simulink model "SecRwLtStRclCmdSrvCal"  (R2018b)
settings: Solver=FixedStepDiscrete  StartTime=0.0  StopTime=10.0  FixedStep=0.01  RelTol=1e-3
undefined symbols (not defined in the file or in its folder): KeSMSwPosInvalidVal_Val, PowerMode1
settings Model: Creator=sn2xws  LastModifiedBy=sn2xws
settings Model: ModifiedHistory=|
  | 2024.5.6
  | V3.0.0 增加零重力电机
  | 2024.8.16 2LZero不动作问题修复
settings DataIOCC: SaveFormat=StructureWithTime
settings OptimizationCC: DefaultParameterBehavior=Inlined  EnhancedBackFolding=on  PassReuseOutputArgsAs=Individual arguments  ZeroExternalMemoryAtStartup=off  ZeroInternalMemoryAtStartup=off  OptimizeBlockOrder=speed  DifferentSizesBufferReuse=on  OptimizationCustomize=off
settings DebuggingCC: ParameterTunabilityLossMsg=error
settings ModelReferenceCC: ModelReferenceNumInstancesAllowed=Single
settings SFSimCC: MATLABDynamicMemAlloc=off
settings RTWCC: SystemTargetFile=autosar.tlc  GenCodeOnly=on  TemplateMakefile=ert_default_tmf  Description=AUTOSAR  GenerateReport=on  IncludeHyperlinkInReport=on  LaunchReport=on  GenerateTraceInfo=on  GenerateTraceReport=on  GenerateTraceReportSl=on  GenerateTraceReportSf=on  GenerateTraceReportEml=on  GenerateCodeMetricsReport=on
settings CodeAppCC: ForceParamTrailComments=on  IgnoreCustomStorageClasses=off  OperatorAnnotations=on  SimulinkDataObjDesc=on  SFDataObjDesc=on  InsertBlockDesc=on
settings STFCustomTargetCC: TargetLangStandard=C99 (ISO)  MultiwordLength=256  ParMdlRefBuildCompliant=on  CompOptLevelCompliant=on  IncludeMdlTerminateFcn=off  CombineOutputUpdateFcns=on  SuppressErrorStatus=on  ERTCustomFileBanners=on  SupportNonFinite=off  SupportComplex=off  SupportContinuousTime=off  SupportNonInlinedSFcns=off  RemoveResetFunc=on  MATLABClassNameForMDSCustomization=Simulink.SoftwareTarget.ERTCustomization  AutosarCompliant=on  UseToolchainInfoCompliant=on  LookupTableObjectStructAxisOrder=2,1,3,4,...  LUTObjectStructOrderEvenSpacing=Size,Table,Breakpoints  SystemTargetFile=autosar.tlc
settings ERTTargetCC: TargetLangStandard=C99 (ISO)  ConcurrentExecutionCompliant=off  IncludeMdlTerminateFcn=off  SuppressErrorStatus=on  SupportNonFinite=off  SupportComplex=off  ModelStepFunctionPrototypeControlCompliant=off  CPPClassGenCompliant=off  AutosarCompliant=on  LookupTableObjectStructAxisOrder=2,1,3,4,...  LUTObjectStructOrderEvenSpacing=Size,Table,Breakpoints  InlinedParameterPlacement=NonHierarchical  ERTCustomFileTemplate=example_file_process.tlc  ERTFilePackagingFormat=Compact

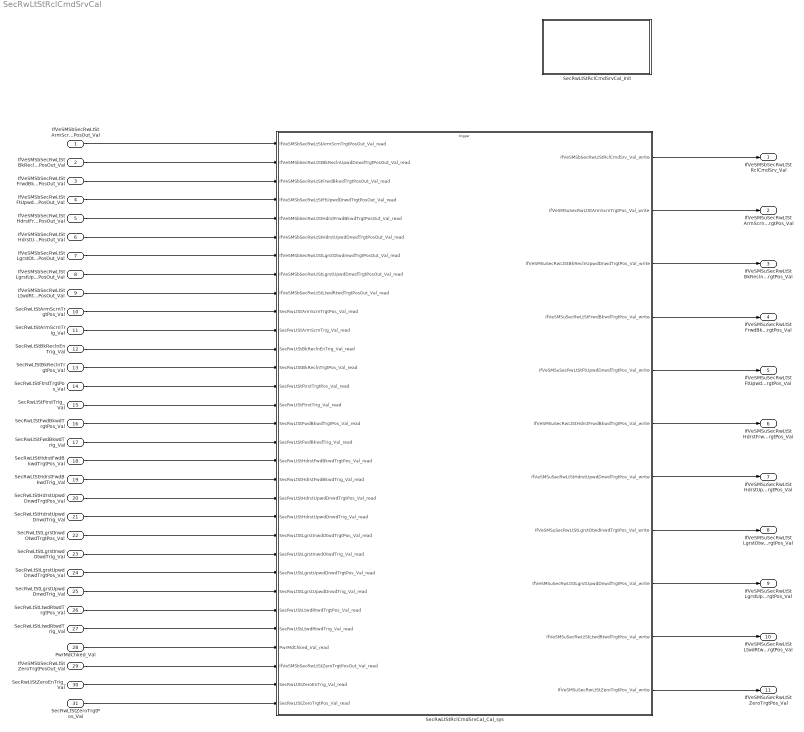
== system SecRwLtStRclCmdSrvCal ==
  IfVeSMSbSecRwLtStArmScrnTrgtPosOut_Val : Inport  OutDataTypeStr=boolean  PortDimensions=1
  IfVeSMSbSecRwLtStBkReclnUpwdDnwdTrgtPosOut_Val : Inport  Port=2  OutDataTypeStr=boolean  PortDimensions=1
  IfVeSMSbSecRwLtStFrwdBkwdTrgtPosOut_Val : Inport  Port=3  OutDataTypeStr=boolean  PortDimensions=1
  IfVeSMSbSecRwLtStFtUpwdDnwdTrgtPosOut_Val : Inport  Port=4  OutDataTypeStr=boolean  PortDimensions=1
  IfVeSMSbSecRwLtStHdrstFrwdBkwdTrgtPosOut_Val : Inport  Port=5  OutDataTypeStr=boolean  PortDimensions=1
  IfVeSMSbSecRwLtStHdrstUpwdDnwdTrgtPosOut_Val : Inport  Port=6  OutDataTypeStr=boolean  PortDimensions=1
  IfVeSMSbSecRwLtStLgrstOtwdInwdTrgtPosOut_Val : Inport  Port=7  OutDataTypeStr=boolean  PortDimensions=1
  IfVeSMSbSecRwLtStLgrstUpwdDnwdTrgtPosOut_Val : Inport  Port=8  OutDataTypeStr=boolean  PortDimensions=1
  IfVeSMSbSecRwLtStLtwdRtwdTrgtPosOut_Val : Inport  Port=9  OutDataTypeStr=boolean  PortDimensions=1
  SecRwLtStArmScrnTrgtPos_Val : Inport  Port=10  OutDataTypeStr=uint16  PortDimensions=1
  SecRwLtStArmScrnTrig_Val : Inport  Port=11  OutDataTypeStr=boolean  PortDimensions=1
  SecRwLtStBkReclnEnTrig_Val : Inport  Port=12  OutDataTypeStr=boolean  PortDimensions=1
  SecRwLtStBkReclnTrgtPos_Val : Inport  Port=13  OutDataTypeStr=uint16  PortDimensions=1
  SecRwLtStFtrstTrgtPos_Val : Inport  Port=14  OutDataTypeStr=uint16  PortDimensions=1
  SecRwLtStFtrstTrig_Val : Inport  Port=15  OutDataTypeStr=boolean  PortDimensions=1
  SecRwLtStFwdBkwdTrgtPos_Val : Inport  Port=16  OutDataTypeStr=uint16  PortDimensions=1
  SecRwLtStFwdBkwdTrig_Val : Inport  Port=17  OutDataTypeStr=boolean  PortDimensions=1
  SecRwLtStHdrstFwdBkwdTrgtPos_Val : Inport  Port=18  OutDataTypeStr=uint16  PortDimensions=1
  SecRwLtStHdrstFwdBkwdTrig_Val : Inport  Port=19  OutDataTypeStr=boolean  PortDimensions=1
  SecRwLtStHdrstUpwdDnwdTrgtPos_Val : Inport  Port=20  OutDataTypeStr=uint16  PortDimensions=1
  SecRwLtStHdrstUpwdDnwdTrig_Val : Inport  Port=21  OutDataTypeStr=boolean  PortDimensions=1
  SecRwLtStLgrstInwdOtwdTrgtPos_Val : Inport  Port=22  OutDataTypeStr=uint16  PortDimensions=1
  SecRwLtStLgrstInwdOtwdTrig_Val : Inport  Port=23  OutDataTypeStr=boolean  PortDimensions=1
  SecRwLtStLgrstUpwdDnwdTrgtPos_Val : Inport  Port=24  OutDataTypeStr=uint16  PortDimensions=1
  SecRwLtStLgrstUpwdDnwdTrig_Val : Inport  Port=25  OutDataTypeStr=boolean  PortDimensions=1
  SecRwLtStLtwdRtwdTrgtPos_Val : Inport  Port=26  OutDataTypeStr=uint16  PortDimensions=1
  SecRwLtStLtwdRtwdTrig_Val : Inport  Port=27  OutDataTypeStr=boolean  PortDimensions=1
  PwrMdChked_Val : Inport  Port=28  OutDataTypeStr=Enum: PowerMode1  PortDimensions=1
  IfVeSMSbSecRwLtStZeroTrgtPosOut_Val : Inport  Port=29  OutDataTypeStr=boolean  PortDimensions=1
  SecRwLtStZeroEnTrig_Val : Inport  Port=30  OutDataTypeStr=boolean  PortDimensions=1
  SecRwLtStZeroTrgtPos_Val : Inport  Port=31  OutDataTypeStr=uint16  PortDimensions=1
  SecRwLtStRclCmdSrvCal_Cal_sys : Subsystem
  SecRwLtStRclCmdSrvCal_Init : Subsystem
  IfVeSMSbSecRwLtStRclCmdSrv_Val : Outport  OutDataTypeStr=boolean  PortDimensions=1
  IfVeSMSuSecRwLtStArmScrnTrgtPos_Val : Outport  Port=2  OutDataTypeStr=uint16  PortDimensions=1
  IfVeSMSuSecRwLtStBkReclnUpwdDnwdTrgtPos_Val : Outport  Port=3  OutDataTypeStr=uint16  PortDimensions=1
  IfVeSMSuSecRwLtStFrwdBkwdTrgtPos_Val : Outport  Port=4  OutDataTypeStr=uint16  PortDimensions=1
  IfVeSMSuSecRwLtStFtUpwdDnwdTrgtPos_Val : Outport  Port=5  OutDataTypeStr=uint16  PortDimensions=1
  IfVeSMSuSecRwLtStHdrstFrwdBkwdTrgtPos_Val : Outport  Port=6  OutDataTypeStr=uint16  PortDimensions=1
  IfVeSMSuSecRwLtStHdrstUpwdDnwdTrgtPos_Val : Outport  Port=7  OutDataTypeStr=uint16  PortDimensions=1
  IfVeSMSuSecRwLtStLgrstOtwdInwdTrgtPos_Val : Outport  Port=8  OutDataTypeStr=uint16  PortDimensions=1
  IfVeSMSuSecRwLtStLgrstUpwdDnwdTrgtPos_Val : Outport  Port=9  OutDataTypeStr=uint16  PortDimensions=1
  IfVeSMSuSecRwLtStLtwdRtwdTrgtPos_Val : Outport  Port=10  OutDataTypeStr=uint16  PortDimensions=1
  IfVeSMSuSecRwLtStZeroTrgtPos_Val : Outport  Port=11  OutDataTypeStr=uint16  PortDimensions=1
  wires:
  IfVeSMSbSecRwLtStArmScrnTrgtPosOut_Val/1 -> SecRwLtStRclCmdSrvCal_Cal_sys/1(IfVeSMSbSecRwLtStArmScrnTrgtPosOut_Val_read)
  IfVeSMSbSecRwLtStBkReclnUpwdDnwdTrgtPosOut_Val/1 -> SecRwLtStRclCmdSrvCal_Cal_sys/2(IfVeSMSbSecRwLtStBkReclnUpwdDnwdTrgtPosOut_Val_read)
  IfVeSMSbSecRwLtStFrwdBkwdTrgtPosOut_Val/1 -> SecRwLtStRclCmdSrvCal_Cal_sys/3(IfVeSMSbSecRwLtStFrwdBkwdTrgtPosOut_Val_read)
  IfVeSMSbSecRwLtStFtUpwdDnwdTrgtPosOut_Val/1 -> SecRwLtStRclCmdSrvCal_Cal_sys/4(IfVeSMSbSecRwLtStFtUpwdDnwdTrgtPosOut_Val_read)
  IfVeSMSbSecRwLtStHdrstFrwdBkwdTrgtPosOut_Val/1 -> SecRwLtStRclCmdSrvCal_Cal_sys/5(IfVeSMSbSecRwLtStHdrstFrwdBkwdTrgtPosOut_Val_read)
  IfVeSMSbSecRwLtStHdrstUpwdDnwdTrgtPosOut_Val/1 -> SecRwLtStRclCmdSrvCal_Cal_sys/6(IfVeSMSbSecRwLtStHdrstUpwdDnwdTrgtPosOut_Val_read)
  IfVeSMSbSecRwLtStLgrstOtwdInwdTrgtPosOut_Val/1 -> SecRwLtStRclCmdSrvCal_Cal_sys/7(IfVeSMSbSecRwLtStLgrstOtwdInwdTrgtPosOut_Val_read)
  IfVeSMSbSecRwLtStLgrstUpwdDnwdTrgtPosOut_Val/1 -> SecRwLtStRclCmdSrvCal_Cal_sys/8(IfVeSMSbSecRwLtStLgrstUpwdDnwdTrgtPosOut_Val_read)
  IfVeSMSbSecRwLtStLtwdRtwdTrgtPosOut_Val/1 -> SecRwLtStRclCmdSrvCal_Cal_sys/9(IfVeSMSbSecRwLtStLtwdRtwdTrgtPosOut_Val_read)
  SecRwLtStArmScrnTrgtPos_Val/1 -> SecRwLtStRclCmdSrvCal_Cal_sys/10(SecRwLtStArmScrnTrgtPos_Val_read)
  SecRwLtStArmScrnTrig_Val/1 -> SecRwLtStRclCmdSrvCal_Cal_sys/11(SecRwLtStArmScrnTrig_Val_read)
  SecRwLtStBkReclnEnTrig_Val/1 -> SecRwLtStRclCmdSrvCal_Cal_sys/12(SecRwLtStBkReclnEnTrig_Val_read)
  SecRwLtStBkReclnTrgtPos_Val/1 -> SecRwLtStRclCmdSrvCal_Cal_sys/13(SecRwLtStBkReclnTrgtPos_Val_read)
  SecRwLtStFtrstTrgtPos_Val/1 -> SecRwLtStRclCmdSrvCal_Cal_sys/14(SecRwLtStFtrstTrgtPos_Val_read)
  SecRwLtStFtrstTrig_Val/1 -> SecRwLtStRclCmdSrvCal_Cal_sys/15(SecRwLtStFtrstTrig_Val_read)
  SecRwLtStFwdBkwdTrgtPos_Val/1 -> SecRwLtStRclCmdSrvCal_Cal_sys/16(SecRwLtStFwdBkwdTrgtPos_Val_read)
  SecRwLtStFwdBkwdTrig_Val/1 -> SecRwLtStRclCmdSrvCal_Cal_sys/17(SecRwLtStFwdBkwdTrig_Val_read)
  SecRwLtStHdrstFwdBkwdTrgtPos_Val/1 -> SecRwLtStRclCmdSrvCal_Cal_sys/18(SecRwLtStHdrstFwdBkwdTrgtPos_Val_read)
  SecRwLtStHdrstFwdBkwdTrig_Val/1 -> SecRwLtStRclCmdSrvCal_Cal_sys/19(SecRwLtStHdrstFwdBkwdTrig_Val_read)
  SecRwLtStHdrstUpwdDnwdTrgtPos_Val/1 -> SecRwLtStRclCmdSrvCal_Cal_sys/20(SecRwLtStHdrstUpwdDnwdTrgtPos_Val_read)
  SecRwLtStHdrstUpwdDnwdTrig_Val/1 -> SecRwLtStRclCmdSrvCal_Cal_sys/21(SecRwLtStHdrstUpwdDnwdTrig_Val_read)
  SecRwLtStLgrstInwdOtwdTrgtPos_Val/1 -> SecRwLtStRclCmdSrvCal_Cal_sys/22(SecRwLtStLgrstInwdOtwdTrgtPos_Val_read)
  SecRwLtStLgrstInwdOtwdTrig_Val/1 -> SecRwLtStRclCmdSrvCal_Cal_sys/23(SecRwLtStLgrstInwdOtwdTrig_Val_read)
  SecRwLtStLgrstUpwdDnwdTrgtPos_Val/1 -> SecRwLtStRclCmdSrvCal_Cal_sys/24(SecRwLtStLgrstUpwdDnwdTrgtPos_Val_read)
  SecRwLtStLgrstUpwdDnwdTrig_Val/1 -> SecRwLtStRclCmdSrvCal_Cal_sys/25(SecRwLtStLgrstUpwdDnwdTrig_Val_read)
  SecRwLtStLtwdRtwdTrgtPos_Val/1 -> SecRwLtStRclCmdSrvCal_Cal_sys/26(SecRwLtStLtwdRtwdTrgtPos_Val_read)
  SecRwLtStLtwdRtwdTrig_Val/1 -> SecRwLtStRclCmdSrvCal_Cal_sys/27(SecRwLtStLtwdRtwdTrig_Val_read)
  SecRwLtStRclCmdSrvCal_Cal_sys/1(IfVeSMSbSecRwLtStRclCmdSrv_Val_write) -> IfVeSMSbSecRwLtStRclCmdSrv_Val/1
  SecRwLtStRclCmdSrvCal_Cal_sys/2(IfVeSMSuSecRwLtStArmScrnTrgtPos_Val_write) -> IfVeSMSuSecRwLtStArmScrnTrgtPos_Val/1
  SecRwLtStRclCmdSrvCal_Cal_sys/3(IfVeSMSuSecRwLtStBkReclnUpwdDnwdTrgtPos_Val_write) -> IfVeSMSuSecRwLtStBkReclnUpwdDnwdTrgtPos_Val/1
  SecRwLtStRclCmdSrvCal_Cal_sys/4(IfVeSMSuSecRwLtStFrwdBkwdTrgtPos_Val_write) -> IfVeSMSuSecRwLtStFrwdBkwdTrgtPos_Val/1
  SecRwLtStRclCmdSrvCal_Cal_sys/5(IfVeSMSuSecRwLtStFtUpwdDnwdTrgtPos_Val_write) -> IfVeSMSuSecRwLtStFtUpwdDnwdTrgtPos_Val/1
  SecRwLtStRclCmdSrvCal_Cal_sys/6(IfVeSMSuSecRwLtStHdrstFrwdBkwdTrgtPos_Val_write) -> IfVeSMSuSecRwLtStHdrstFrwdBkwdTrgtPos_Val/1
  SecRwLtStRclCmdSrvCal_Cal_sys/7(IfVeSMSuSecRwLtStHdrstUpwdDnwdTrgtPos_Val_write) -> IfVeSMSuSecRwLtStHdrstUpwdDnwdTrgtPos_Val/1
  SecRwLtStRclCmdSrvCal_Cal_sys/8(IfVeSMSuSecRwLtStLgrstOtwdInwdTrgtPos_Val_write) -> IfVeSMSuSecRwLtStLgrstOtwdInwdTrgtPos_Val/1
  SecRwLtStRclCmdSrvCal_Cal_sys/9(IfVeSMSuSecRwLtStLgrstUpwdDnwdTrgtPos_Val_write) -> IfVeSMSuSecRwLtStLgrstUpwdDnwdTrgtPos_Val/1
  SecRwLtStRclCmdSrvCal_Cal_sys/10(IfVeSMSuSecRwLtStLtwdRtwdTrgtPos_Val_write) -> IfVeSMSuSecRwLtStLtwdRtwdTrgtPos_Val/1
  PwrMdChked_Val/1 -> SecRwLtStRclCmdSrvCal_Cal_sys/28(PwrMdChked_Val_read)
  IfVeSMSbSecRwLtStZeroTrgtPosOut_Val/1 -> SecRwLtStRclCmdSrvCal_Cal_sys/29(IfVeSMSbSecRwLtStZeroTrgtPosOut_Val_read)
  SecRwLtStZeroEnTrig_Val/1 -> SecRwLtStRclCmdSrvCal_Cal_sys/30(SecRwLtStZeroEnTrig_Val_read)
  SecRwLtStZeroTrgtPos_Val/1 -> SecRwLtStRclCmdSrvCal_Cal_sys/31(SecRwLtStZeroTrgtPos_Val_read)
  SecRwLtStRclCmdSrvCal_Cal_sys/11(IfVeSMSuSecRwLtStZeroTrgtPos_Val_write) -> IfVeSMSuSecRwLtStZeroTrgtPos_Val/1

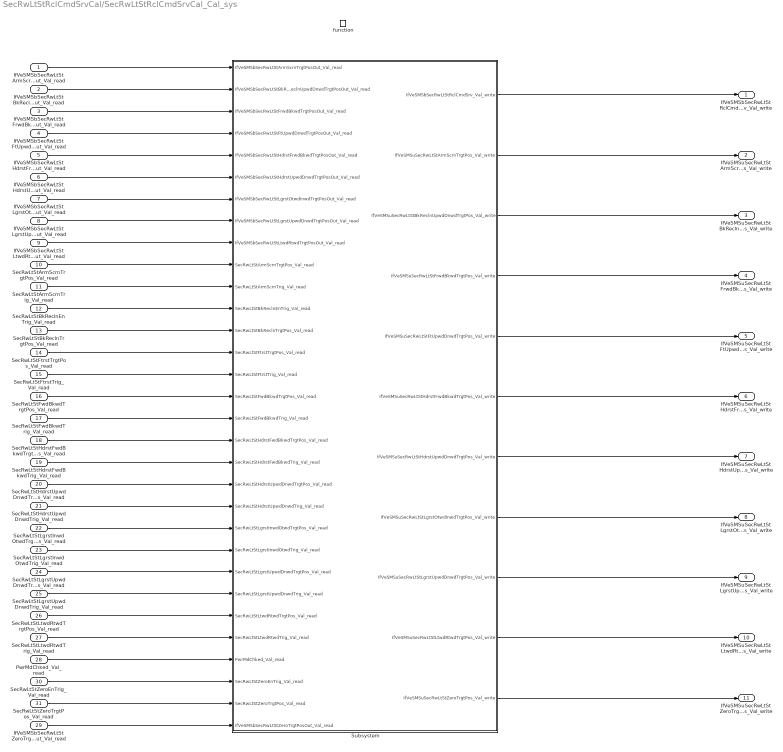
== system SecRwLtStRclCmdSrvCal/SecRwLtStRclCmdSrvCal_Cal_sys ==
  IfVeSMSbSecRwLtStArmScrnTrgtPosOut_Val_read : Inport
  IfVeSMSbSecRwLtStBkReclnUpwdDnwdTrgtPosOut_Val_read : Inport  Port=2
  IfVeSMSbSecRwLtStFrwdBkwdTrgtPosOut_Val_read : Inport  Port=3
  IfVeSMSbSecRwLtStFtUpwdDnwdTrgtPosOut_Val_read : Inport  Port=4
  IfVeSMSbSecRwLtStHdrstFrwdBkwdTrgtPosOut_Val_read : Inport  Port=5
  IfVeSMSbSecRwLtStHdrstUpwdDnwdTrgtPosOut_Val_read : Inport  Port=6
  IfVeSMSbSecRwLtStLgrstOtwdInwdTrgtPosOut_Val_read : Inport  Port=7
  IfVeSMSbSecRwLtStLgrstUpwdDnwdTrgtPosOut_Val_read : Inport  Port=8
  IfVeSMSbSecRwLtStLtwdRtwdTrgtPosOut_Val_read : Inport  Port=9
  SecRwLtStArmScrnTrgtPos_Val_read : Inport  Port=10
  SecRwLtStArmScrnTrig_Val_read : Inport  Port=11
  SecRwLtStBkReclnEnTrig_Val_read : Inport  Port=12
  SecRwLtStBkReclnTrgtPos_Val_read : Inport  Port=13
  SecRwLtStFtrstTrgtPos_Val_read : Inport  Port=14
  SecRwLtStFtrstTrig_Val_read : Inport  Port=15
  SecRwLtStFwdBkwdTrgtPos_Val_read : Inport  Port=16
  SecRwLtStFwdBkwdTrig_Val_read : Inport  Port=17
  SecRwLtStHdrstFwdBkwdTrgtPos_Val_read : Inport  Port=18
  SecRwLtStHdrstFwdBkwdTrig_Val_read : Inport  Port=19
  SecRwLtStHdrstUpwdDnwdTrgtPos_Val_read : Inport  Port=20
  SecRwLtStHdrstUpwdDnwdTrig_Val_read : Inport  Port=21
  SecRwLtStLgrstInwdOtwdTrgtPos_Val_read : Inport  Port=22
  SecRwLtStLgrstInwdOtwdTrig_Val_read : Inport  Port=23
  SecRwLtStLgrstUpwdDnwdTrgtPos_Val_read : Inport  Port=24
  SecRwLtStLgrstUpwdDnwdTrig_Val_read : Inport  Port=25
  SecRwLtStLtwdRtwdTrgtPos_Val_read : Inport  Port=26
  SecRwLtStLtwdRtwdTrig_Val_read : Inport  Port=27
  PwrMdChked_Val_read : Inport  Port=28
  IfVeSMSbSecRwLtStZeroTrgtPosOut_Val_read : Inport  Port=29
  SecRwLtStZeroEnTrig_Val_read : Inport  Port=30
  SecRwLtStZeroTrgtPos_Val_read : Inport  Port=31
  function : TriggerPort  TriggerType=function-call  IsSimulinkFunction=on  FunctionName=SecRwLtStRclCmdSrvCal_Cal  VariantControl=(inherit)
  Subsystem : Subsystem
  IfVeSMSbSecRwLtStRclCmdSrv_Val_write : Outport
      settings: EnsureOutportIsVirtual=on
  IfVeSMSuSecRwLtStArmScrnTrgtPos_Val_write : Outport  Port=2
      settings: EnsureOutportIsVirtual=on
  IfVeSMSuSecRwLtStBkReclnUpwdDnwdTrgtPos_Val_write : Outport  Port=3
      settings: EnsureOutportIsVirtual=on
  IfVeSMSuSecRwLtStFrwdBkwdTrgtPos_Val_write : Outport  Port=4
      settings: EnsureOutportIsVirtual=on
  IfVeSMSuSecRwLtStFtUpwdDnwdTrgtPos_Val_write : Outport  Port=5
      settings: EnsureOutportIsVirtual=on
  IfVeSMSuSecRwLtStHdrstFrwdBkwdTrgtPos_Val_write : Outport  Port=6
      settings: EnsureOutportIsVirtual=on
  IfVeSMSuSecRwLtStHdrstUpwdDnwdTrgtPos_Val_write : Outport  Port=7
      settings: EnsureOutportIsVirtual=on
  IfVeSMSuSecRwLtStLgrstOtwdInwdTrgtPos_Val_write : Outport  Port=8
      settings: EnsureOutportIsVirtual=on
  IfVeSMSuSecRwLtStLgrstUpwdDnwdTrgtPos_Val_write : Outport  Port=9
      settings: EnsureOutportIsVirtual=on
  IfVeSMSuSecRwLtStLtwdRtwdTrgtPos_Val_write : Outport  Port=10
      settings: EnsureOutportIsVirtual=on
  IfVeSMSuSecRwLtStZeroTrgtPos_Val_write : Outport  Port=11
      settings: EnsureOutportIsVirtual=on
  wires:
  IfVeSMSbSecRwLtStHdrstUpwdDnwdTrgtPosOut_Val_read/1 -> Subsystem/6(IfVeSMSbSecRwLtStHdrstUpwdDnwdTrgtPosOut_Val_read)
  IfVeSMSbSecRwLtStLgrstOtwdInwdTrgtPosOut_Val_read/1 -> Subsystem/7(IfVeSMSbSecRwLtStLgrstOtwdInwdTrgtPosOut_Val_read)
  IfVeSMSbSecRwLtStLgrstUpwdDnwdTrgtPosOut_Val_read/1 -> Subsystem/8(IfVeSMSbSecRwLtStLgrstUpwdDnwdTrgtPosOut_Val_read)
  IfVeSMSbSecRwLtStFtUpwdDnwdTrgtPosOut_Val_read/1 -> Subsystem/4(IfVeSMSbSecRwLtStFtUpwdDnwdTrgtPosOut_Val_read)
  IfVeSMSbSecRwLtStHdrstFrwdBkwdTrgtPosOut_Val_read/1 -> Subsystem/5(IfVeSMSbSecRwLtStHdrstFrwdBkwdTrgtPosOut_Val_read)
  IfVeSMSbSecRwLtStLtwdRtwdTrgtPosOut_Val_read/1 -> Subsystem/9(IfVeSMSbSecRwLtStLtwdRtwdTrgtPosOut_Val_read)
  SecRwLtStArmScrnTrgtPos_Val_read/1 -> Subsystem/10(SecRwLtStArmScrnTrgtPos_Val_read)
  IfVeSMSbSecRwLtStArmScrnTrgtPosOut_Val_read/1 -> Subsystem/1(IfVeSMSbSecRwLtStArmScrnTrgtPosOut_Val_read)
  IfVeSMSbSecRwLtStBkReclnUpwdDnwdTrgtPosOut_Val_read/1 -> Subsystem/2(IfVeSMSbSecRwLtStBkReclnUpwdDnwdTrgtPosOut_Val_read)
  IfVeSMSbSecRwLtStFrwdBkwdTrgtPosOut_Val_read/1 -> Subsystem/3(IfVeSMSbSecRwLtStFrwdBkwdTrgtPosOut_Val_read)
  SecRwLtStArmScrnTrig_Val_read/1 -> Subsystem/11(SecRwLtStArmScrnTrig_Val_read)
  SecRwLtStBkReclnEnTrig_Val_read/1 -> Subsystem/12(SecRwLtStBkReclnEnTrig_Val_read)
  SecRwLtStBkReclnTrgtPos_Val_read/1 -> Subsystem/13(SecRwLtStBkReclnTrgtPos_Val_read)
  SecRwLtStFtrstTrgtPos_Val_read/1 -> Subsystem/14(SecRwLtStFtrstTrgtPos_Val_read)
  SecRwLtStFtrstTrig_Val_read/1 -> Subsystem/15(SecRwLtStFtrstTrig_Val_read)
  SecRwLtStFwdBkwdTrgtPos_Val_read/1 -> Subsystem/16(SecRwLtStFwdBkwdTrgtPos_Val_read)
  SecRwLtStFwdBkwdTrig_Val_read/1 -> Subsystem/17(SecRwLtStFwdBkwdTrig_Val_read)
  SecRwLtStHdrstFwdBkwdTrgtPos_Val_read/1 -> Subsystem/18(SecRwLtStHdrstFwdBkwdTrgtPos_Val_read)
  SecRwLtStHdrstFwdBkwdTrig_Val_read/1 -> Subsystem/19(SecRwLtStHdrstFwdBkwdTrig_Val_read)
  SecRwLtStHdrstUpwdDnwdTrgtPos_Val_read/1 -> Subsystem/20(SecRwLtStHdrstUpwdDnwdTrgtPos_Val_read)
  SecRwLtStHdrstUpwdDnwdTrig_Val_read/1 -> Subsystem/21(SecRwLtStHdrstUpwdDnwdTrig_Val_read)
  SecRwLtStLgrstInwdOtwdTrgtPos_Val_read/1 -> Subsystem/22(SecRwLtStLgrstInwdOtwdTrgtPos_Val_read)
  SecRwLtStLgrstInwdOtwdTrig_Val_read/1 -> Subsystem/23(SecRwLtStLgrstInwdOtwdTrig_Val_read)
  SecRwLtStLgrstUpwdDnwdTrgtPos_Val_read/1 -> Subsystem/24(SecRwLtStLgrstUpwdDnwdTrgtPos_Val_read)
  SecRwLtStLgrstUpwdDnwdTrig_Val_read/1 -> Subsystem/25(SecRwLtStLgrstUpwdDnwdTrig_Val_read)
  SecRwLtStLtwdRtwdTrgtPos_Val_read/1 -> Subsystem/26(SecRwLtStLtwdRtwdTrgtPos_Val_read)
  SecRwLtStLtwdRtwdTrig_Val_read/1 -> Subsystem/27(SecRwLtStLtwdRtwdTrig_Val_read)
  Subsystem/1(IfVeSMSbSecRwLtStRclCmdSrv_Val_write) -> IfVeSMSbSecRwLtStRclCmdSrv_Val_write/1
  Subsystem/2(IfVeSMSuSecRwLtStArmScrnTrgtPos_Val_write) -> IfVeSMSuSecRwLtStArmScrnTrgtPos_Val_write/1
  Subsystem/3(IfVeSMSuSecRwLtStBkReclnUpwdDnwdTrgtPos_Val_write) -> IfVeSMSuSecRwLtStBkReclnUpwdDnwdTrgtPos_Val_write/1
  Subsystem/4(IfVeSMSuSecRwLtStFrwdBkwdTrgtPos_Val_write) -> IfVeSMSuSecRwLtStFrwdBkwdTrgtPos_Val_write/1
  Subsystem/5(IfVeSMSuSecRwLtStFtUpwdDnwdTrgtPos_Val_write) -> IfVeSMSuSecRwLtStFtUpwdDnwdTrgtPos_Val_write/1
  Subsystem/6(IfVeSMSuSecRwLtStHdrstFrwdBkwdTrgtPos_Val_write) -> IfVeSMSuSecRwLtStHdrstFrwdBkwdTrgtPos_Val_write/1
  Subsystem/7(IfVeSMSuSecRwLtStHdrstUpwdDnwdTrgtPos_Val_write) -> IfVeSMSuSecRwLtStHdrstUpwdDnwdTrgtPos_Val_write/1
  Subsystem/8(IfVeSMSuSecRwLtStLgrstOtwdInwdTrgtPos_Val_write) -> IfVeSMSuSecRwLtStLgrstOtwdInwdTrgtPos_Val_write/1
  Subsystem/9(IfVeSMSuSecRwLtStLgrstUpwdDnwdTrgtPos_Val_write) -> IfVeSMSuSecRwLtStLgrstUpwdDnwdTrgtPos_Val_write/1
  Subsystem/10(IfVeSMSuSecRwLtStLtwdRtwdTrgtPos_Val_write) -> IfVeSMSuSecRwLtStLtwdRtwdTrgtPos_Val_write/1
  PwrMdChked_Val_read/1 -> Subsystem/28(PwrMdChked_Val_read)
  Subsystem/11(IfVeSMSuSecRwLtStZeroTrgtPos_Val_write) -> IfVeSMSuSecRwLtStZeroTrgtPos_Val_write/1
  SecRwLtStZeroEnTrig_Val_read/1 -> Subsystem/29(SecRwLtStZeroEnTrig_Val_read)
  SecRwLtStZeroTrgtPos_Val_read/1 -> Subsystem/30(SecRwLtStZeroTrgtPos_Val_read)
  IfVeSMSbSecRwLtStZeroTrgtPosOut_Val_read/1 -> Subsystem/31(IfVeSMSbSecRwLtStZeroTrgtPosOut_Val_read)

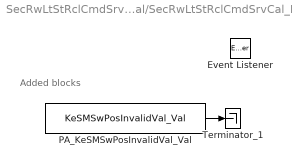
== system SecRwLtStRclCmdSrvCal/SecRwLtStRclCmdSrvCal_Init ==
  note: Added blocks
  Event Listener : EventListener  EventName=reset
  PA_KeSMSwPosInvalidVal_Val : Constant  Value=KeSMSwPosInvalidVal_Val
  Terminator_1 : Terminator
  wires:
  PA_KeSMSwPosInvalidVal_Val/1 -> Terminator_1/1

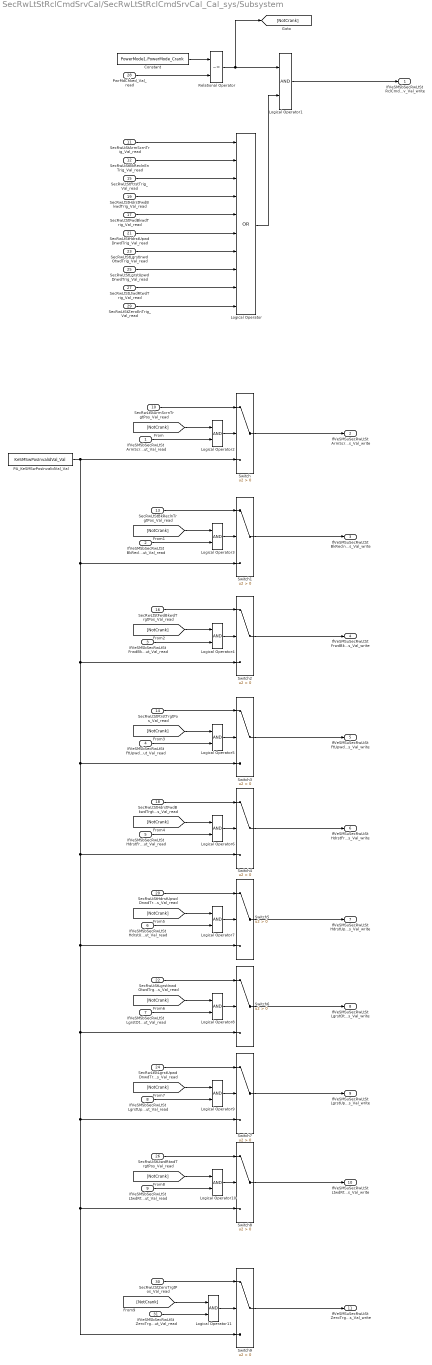
== system SecRwLtStRclCmdSrvCal/SecRwLtStRclCmdSrvCal_Cal_sys/Subsystem ==
  IfVeSMSbSecRwLtStArmScrnTrgtPosOut_Val_read : Inport
  IfVeSMSbSecRwLtStBkReclnUpwdDnwdTrgtPosOut_Val_read : Inport  Port=2
  IfVeSMSbSecRwLtStFrwdBkwdTrgtPosOut_Val_read : Inport  Port=3
  IfVeSMSbSecRwLtStFtUpwdDnwdTrgtPosOut_Val_read : Inport  Port=4
  IfVeSMSbSecRwLtStHdrstFrwdBkwdTrgtPosOut_Val_read : Inport  Port=5
  IfVeSMSbSecRwLtStHdrstUpwdDnwdTrgtPosOut_Val_read : Inport  Port=6
  IfVeSMSbSecRwLtStLgrstOtwdInwdTrgtPosOut_Val_read : Inport  Port=7
  IfVeSMSbSecRwLtStLgrstUpwdDnwdTrgtPosOut_Val_read : Inport  Port=8
  IfVeSMSbSecRwLtStLtwdRtwdTrgtPosOut_Val_read : Inport  Port=9
  SecRwLtStArmScrnTrgtPos_Val_read : Inport  Port=10
  SecRwLtStArmScrnTrig_Val_read : Inport  Port=11
  SecRwLtStBkReclnEnTrig_Val_read : Inport  Port=12
  SecRwLtStBkReclnTrgtPos_Val_read : Inport  Port=13
  SecRwLtStFtrstTrgtPos_Val_read : Inport  Port=14
  SecRwLtStFtrstTrig_Val_read : Inport  Port=15
  SecRwLtStFwdBkwdTrgtPos_Val_read : Inport  Port=16
  SecRwLtStFwdBkwdTrig_Val_read : Inport  Port=17
  SecRwLtStHdrstFwdBkwdTrgtPos_Val_read : Inport  Port=18
  SecRwLtStHdrstFwdBkwdTrig_Val_read : Inport  Port=19
  SecRwLtStHdrstUpwdDnwdTrgtPos_Val_read : Inport  Port=20
  SecRwLtStHdrstUpwdDnwdTrig_Val_read : Inport  Port=21
  SecRwLtStLgrstInwdOtwdTrgtPos_Val_read : Inport  Port=22
  SecRwLtStLgrstInwdOtwdTrig_Val_read : Inport  Port=23
  SecRwLtStLgrstUpwdDnwdTrgtPos_Val_read : Inport  Port=24
  SecRwLtStLgrstUpwdDnwdTrig_Val_read : Inport  Port=25
  SecRwLtStLtwdRtwdTrgtPos_Val_read : Inport  Port=26
  SecRwLtStLtwdRtwdTrig_Val_read : Inport  Port=27
  PwrMdChked_Val_read : Inport  Port=28
  SecRwLtStZeroEnTrig_Val_read : Inport  Port=29
  SecRwLtStZeroTrgtPos_Val_read : Inport  Port=30
  IfVeSMSbSecRwLtStZeroTrgtPosOut_Val_read : Inport  Port=31
  Constant : Constant  Value=PowerMode1.PowerMode_Crank  OutDataTypeStr=Enum: PowerMode1
  Logical Operator : Logic  Operator=OR  Inputs=10  AllPortsSameDT=off  OutDataTypeStr=boolean
  Logical Operator{1..11} (11 alike) : Logic  AllPortsSameDT=off  OutDataTypeStr=boolean
  PA_KeSMSwPosInvalidVal_Val : Constant  Value=KeSMSwPosInvalidVal_Val
  Relational Operator : RelationalOperator  Operator=~=  OutDataTypeStr=boolean  RndMeth=Simplest
  Switch{,1..9} (10 alike) : Switch  Criteria=u2 > Threshold
  IfVeSMSbSecRwLtStRclCmdSrv_Val_write : Outport
      settings: EnsureOutportIsVirtual=on
  IfVeSMSuSecRwLtStArmScrnTrgtPos_Val_write : Outport  Port=2
      settings: EnsureOutportIsVirtual=on
  IfVeSMSuSecRwLtStBkReclnUpwdDnwdTrgtPos_Val_write : Outport  Port=3
      settings: EnsureOutportIsVirtual=on
  IfVeSMSuSecRwLtStFrwdBkwdTrgtPos_Val_write : Outport  Port=4
      settings: EnsureOutportIsVirtual=on
  IfVeSMSuSecRwLtStFtUpwdDnwdTrgtPos_Val_write : Outport  Port=5
      settings: EnsureOutportIsVirtual=on
  IfVeSMSuSecRwLtStHdrstFrwdBkwdTrgtPos_Val_write : Outport  Port=6
      settings: EnsureOutportIsVirtual=on
  IfVeSMSuSecRwLtStHdrstUpwdDnwdTrgtPos_Val_write : Outport  Port=7
      settings: EnsureOutportIsVirtual=on
  IfVeSMSuSecRwLtStLgrstOtwdInwdTrgtPos_Val_write : Outport  Port=8
      settings: EnsureOutportIsVirtual=on
  IfVeSMSuSecRwLtStLgrstUpwdDnwdTrgtPos_Val_write : Outport  Port=9
      settings: EnsureOutportIsVirtual=on
  IfVeSMSuSecRwLtStLtwdRtwdTrgtPos_Val_write : Outport  Port=10
      settings: EnsureOutportIsVirtual=on
  IfVeSMSuSecRwLtStZeroTrgtPos_Val_write : Outport  Port=11
      settings: EnsureOutportIsVirtual=on
  wires:
  SecRwLtStLtwdRtwdTrig_Val_read/1 -> Logical Operator/9
  SecRwLtStArmScrnTrig_Val_read/1 -> Logical Operator/1
  SecRwLtStFwdBkwdTrig_Val_read/1 -> Logical Operator/5
  SecRwLtStLgrstInwdOtwdTrig_Val_read/1 -> Logical Operator/7
  SecRwLtStLgrstUpwdDnwdTrig_Val_read/1 -> Logical Operator/8
  SecRwLtStBkReclnEnTrig_Val_read/1 -> Logical Operator/2
  SecRwLtStHdrstUpwdDnwdTrig_Val_read/1 -> Logical Operator/6
  SecRwLtStFtrstTrig_Val_read/1 -> Logical Operator/3
  SecRwLtStHdrstFwdBkwdTrig_Val_read/1 -> Logical Operator/4
  SecRwLtStArmScrnTrgtPos_Val_read/1 -> Switch/1
  SecRwLtStBkReclnTrgtPos_Val_read/1 -> Switch1/1
  SecRwLtStFtrstTrgtPos_Val_read/1 -> Switch3/1
  SecRwLtStFwdBkwdTrgtPos_Val_read/1 -> Switch2/1
  SecRwLtStHdrstFwdBkwdTrgtPos_Val_read/1 -> Switch4/1
  SecRwLtStHdrstUpwdDnwdTrgtPos_Val_read/1 -> Switch5/1
  SecRwLtStLgrstInwdOtwdTrgtPos_Val_read/1 -> Switch6/1
  SecRwLtStLgrstUpwdDnwdTrgtPos_Val_read/1 -> Switch7/1
  SecRwLtStLtwdRtwdTrgtPos_Val_read/1 -> Switch8/1
  PA_KeSMSwPosInvalidVal_Val/1 -> Switch2/3, Switch9/3, Switch8/3, Switch7/3, Switch6/3, Switch5/3, Switch4/3, Switch3/3, Switch1/3, Switch/3
  Switch/1 -> IfVeSMSuSecRwLtStArmScrnTrgtPos_Val_write/1
  Switch1/1 -> IfVeSMSuSecRwLtStBkReclnUpwdDnwdTrgtPos_Val_write/1
  Switch2/1 -> IfVeSMSuSecRwLtStFrwdBkwdTrgtPos_Val_write/1
  Switch3/1 -> IfVeSMSuSecRwLtStFtUpwdDnwdTrgtPos_Val_write/1
  Switch4/1 -> IfVeSMSuSecRwLtStHdrstFrwdBkwdTrgtPos_Val_write/1
  Switch5/1 -> IfVeSMSuSecRwLtStHdrstUpwdDnwdTrgtPos_Val_write/1
  Switch6/1 -> IfVeSMSuSecRwLtStLgrstOtwdInwdTrgtPos_Val_write/1
  Switch7/1 -> IfVeSMSuSecRwLtStLgrstUpwdDnwdTrgtPos_Val_write/1
  Switch8/1 -> IfVeSMSuSecRwLtStLtwdRtwdTrgtPos_Val_write/1
  PwrMdChked_Val_read/1 -> Relational Operator/2
  Relational Operator/1 -> [NotCrank], Logical Operator1/1
  Logical Operator1/1 -> IfVeSMSbSecRwLtStRclCmdSrv_Val_write/1
  Constant/1 -> Relational Operator/1
  Logical Operator/1 -> Logical Operator1/2
  IfVeSMSbSecRwLtStArmScrnTrgtPosOut_Val_read/1 -> Logical Operator2/2
  [NotCrank] -> Logical Operator2/1
  Logical Operator2/1 -> Switch/2
  [NotCrank] -> Logical Operator3/1
  Logical Operator3/1 -> Switch1/2
  IfVeSMSbSecRwLtStBkReclnUpwdDnwdTrgtPosOut_Val_read/1 -> Logical Operator3/2
  [NotCrank] -> Logical Operator4/1
  Logical Operator4/1 -> Switch2/2
  IfVeSMSbSecRwLtStFrwdBkwdTrgtPosOut_Val_read/1 -> Logical Operator4/2
  [NotCrank] -> Logical Operator5/1
  Logical Operator5/1 -> Switch3/2
  IfVeSMSbSecRwLtStFtUpwdDnwdTrgtPosOut_Val_read/1 -> Logical Operator5/2
  [NotCrank] -> Logical Operator6/1
  Logical Operator6/1 -> Switch4/2
  IfVeSMSbSecRwLtStHdrstFrwdBkwdTrgtPosOut_Val_read/1 -> Logical Operator6/2
  [NotCrank] -> Logical Operator7/1
  Logical Operator7/1 -> Switch5/2
  IfVeSMSbSecRwLtStHdrstUpwdDnwdTrgtPosOut_Val_read/1 -> Logical Operator7/2
  [NotCrank] -> Logical Operator8/1
  Logical Operator8/1 -> Switch6/2
  IfVeSMSbSecRwLtStLgrstOtwdInwdTrgtPosOut_Val_read/1 -> Logical Operator8/2
  [NotCrank] -> Logical Operator9/1
  Logical Operator9/1 -> Switch7/2
  IfVeSMSbSecRwLtStLgrstUpwdDnwdTrgtPosOut_Val_read/1 -> Logical Operator9/2
  [NotCrank] -> Logical Operator10/1
  Logical Operator10/1 -> Switch8/2
  IfVeSMSbSecRwLtStLtwdRtwdTrgtPosOut_Val_read/1 -> Logical Operator10/2
  SecRwLtStZeroEnTrig_Val_read/1 -> Logical Operator/10
  Switch9/1 -> IfVeSMSuSecRwLtStZeroTrgtPos_Val_write/1
  Logical Operator11/1 -> Switch9/2
  [NotCrank] -> Logical Operator11/1
  SecRwLtStZeroTrgtPos_Val_read/1 -> Switch9/1
  IfVeSMSbSecRwLtStZeroTrgtPosOut_Val_read/1 -> Logical Operator11/2
